simulink model "networkanalyzer"  (R2012b)
settings: Solver=ode3  SolverMode=SingleTasking  StartTime=0.0  StopTime=50000  RelTol=1e-3
libraries: xbsIndex_r4 x1097, casper_library_flow_control x33, casper_library_misc x21, xps_library x10
(part 5 of 8)

== system networkanalyzer/DFTMem2/MemRecord ==
  Start : Inport
  DataIn : Inport  Port=2
  WE : Inport  Port=3
  Constant6 : xbsIndex_r4/Constant  const=16383  gui_display_data_type=Fixed-point  arith_type=Unsigned  n_bits=14  bin_pt=0  preci_type=Single  exp_width=8  frac_width=24  explicit_period=off  period=1  equ=P=C  opselect=C  inp2=PCIN>>17  opr=+  inp1=P  carry=CIN  dbl_ovrd=off  block_type=constant
  Delay{,1..3} (4 alike) : xbsIndex_r4/Delay  rst=off  infoeditControl=Selection of Reset will increase slice count due to use of real FFs and instead of SRLs  en=off  latency=1  dbl_ovrd=off  reg_retiming=off  block_type=delay
  Gateway Out{1..6} (6 alike) : xbsIndex_r4/Gateway Out  inherit_from_input=off  hdl_port=off  timing_constraint=None  locs_specified=off  LOCs={}  UseAsDAC=off  DACChannel='1'  block_type=gatewayout
  Logical : xbsIndex_r4/Logical  logical_function=AND  inputs=2  en=off  latency=0  precision=Full  arith_type=Unsigned  n_bits=16  bin_pt=0  align_bp=on  dbl_ovrd=off  block_type=logical
  MCode : xbsIndex_r4/MCode  mfname=viewmemcontrol  explicit_period=on  period=1  inputsTable={'boundInpExpr'=>['start','endcnt','state'],'inputs'=>['start','endcnt','state']}  outputsTable={'outputs'=>['cnten','cntrst','nextstate'],'suppressOut'=>['off','off','off']}  dbl_ovrd=off  enable_stdout=on  enable_debug=off  suppress_output=on  defparams={'start',start,'endcnt',endcnt,'state',state}  hide_port_list={}  block_type=mcode
  Register : xbsIndex_r4/Register  init=0  rst=off  en=off  dbl_ovrd=off  block_type=register
  Relational : xbsIndex_r4/Relational  mode=a=b  en=off  latency=0  dbl_ovrd=off  block_type=relational
  Shared BRAM : Subsystem  Tag=xps:bram  AncestorBlock=xps_library/Shared BRAM  mask{arith_type=Unsigned, addr_width=14, data_width=32, reg_prim_output=off, reg_core_output=off, optimization=Minimum_Area, data_bin_pt=0, init_vals=[0:2^10-1], sample_rate=1}
      mask prompts: arith_type "Output Data Type"; addr_width "Address width"; data_width "Data Width"; reg_prim_output "Register Primitive Output"; reg_core_output "Register Core Output"; data_bin_pt "Data Binary Point"; init_vals "Initial values (simulation only)"; sample_rate "Sample rate"
      mask init:
      | shared_bram_mask;
      mask TypeOptions arith_type: Unsigned | Signed  (2's comp)
      mask TypeOptions data_width: 8 | 16 | 32 | 64 | 128
      mask TypeOptions optimization: Minimum_Area | Low_Power
  Terminator13 : Terminator
  memrecordscope : Scope  NumInputPorts=8
      settings: YMin=0~-5~-5~-5~-5~-5~-5~-5  YMax=300000~5~5~5~5~5~5~5  MaxDataPoints=10000
  spect_cnt : xbsIndex_r4/Counter  cnt_type=Free Running  cnt_to=Inf  operation=Up  start_count=0  cnt_by_val=1  arith_type=Unsigned  n_bits=14  bin_pt=0  load_pin=off  rst=on  en=on  explicit_period=on  period=1  dbl_ovrd=off  use_behavioral_HDL=off  implementation=Fabric  use_rpm=off  block_type=counter
  memDone : Outport
  wires:
  DataIn/1 -> Delay3/1
  Start/1 -> Gateway Out1/1, MCode/1
  spect_cnt/1 -> Relational/2, Gateway Out3/1, Delay1/1
  Delay/1 -> Terminator13/1
  Constant6/1 -> Relational/1
  MCode/2 -> spect_cnt/1
  Relational/1 -> Gateway Out6/1, memDone/1, MCode/2
  Register/1 -> MCode/3, Gateway Out2/1
  MCode/3 -> Register/1
  MCode/1 -> Logical/1
  Logical/1 -> Gateway Out4/1, Delay2/1, spect_cnt/2
  WE/1 -> Logical/2
  Gateway Out5/1 -> memrecordscope/1
  Gateway Out1/1 -> memrecordscope/2
  Gateway Out2/1 -> memrecordscope/3
  Gateway Out3/1 -> memrecordscope/4
  Gateway Out4/1 -> memrecordscope/5
  Gateway Out6/1 -> memrecordscope/6
  Delay1/1 -> Shared BRAM/1(addr)
  Delay3/1 -> Shared BRAM/2(data_in)
  Delay2/1 -> Shared BRAM/3(we)
  Shared BRAM/1(data_out) -> Gateway Out5/1, Delay/1

== system networkanalyzer/DFTMem3/MemRecord ==
  Start : Inport
  DataIn : Inport  Port=2
  WE : Inport  Port=3
  Constant6 : xbsIndex_r4/Constant  const=16383  gui_display_data_type=Fixed-point  arith_type=Unsigned  n_bits=14  bin_pt=0  preci_type=Single  exp_width=8  frac_width=24  explicit_period=off  period=1  equ=P=C  opselect=C  inp2=PCIN>>17  opr=+  inp1=P  carry=CIN  dbl_ovrd=off  block_type=constant
  Delay{,1..3} (4 alike) : xbsIndex_r4/Delay  rst=off  infoeditControl=Selection of Reset will increase slice count due to use of real FFs and instead of SRLs  en=off  latency=1  dbl_ovrd=off  reg_retiming=off  block_type=delay
  Gateway Out{1..6} (6 alike) : xbsIndex_r4/Gateway Out  inherit_from_input=off  hdl_port=off  timing_constraint=None  locs_specified=off  LOCs={}  UseAsDAC=off  DACChannel='1'  block_type=gatewayout
  Logical : xbsIndex_r4/Logical  logical_function=AND  inputs=2  en=off  latency=0  precision=Full  arith_type=Unsigned  n_bits=16  bin_pt=0  align_bp=on  dbl_ovrd=off  block_type=logical
  MCode : xbsIndex_r4/MCode  mfname=viewmemcontrol  explicit_period=on  period=1  inputsTable={'boundInpExpr'=>['start','endcnt','state'],'inputs'=>['start','endcnt','state']}  outputsTable={'outputs'=>['cnten','cntrst','nextstate'],'suppressOut'=>['off','off','off']}  dbl_ovrd=off  enable_stdout=on  enable_debug=off  suppress_output=on  defparams={'start',start,'endcnt',endcnt,'state',state}  hide_port_list={}  block_type=mcode
  Register : xbsIndex_r4/Register  init=0  rst=off  en=off  dbl_ovrd=off  block_type=register
  Relational : xbsIndex_r4/Relational  mode=a=b  en=off  latency=0  dbl_ovrd=off  block_type=relational
  Shared BRAM : Subsystem  Tag=xps:bram  AncestorBlock=xps_library/Shared BRAM  mask{arith_type=Unsigned, addr_width=14, data_width=32, reg_prim_output=off, reg_core_output=off, optimization=Minimum_Area, data_bin_pt=0, init_vals=[0:2^10-1], sample_rate=1}
      mask prompts: arith_type "Output Data Type"; addr_width "Address width"; data_width "Data Width"; reg_prim_output "Register Primitive Output"; reg_core_output "Register Core Output"; data_bin_pt "Data Binary Point"; init_vals "Initial values (simulation only)"; sample_rate "Sample rate"
      mask init:
      | shared_bram_mask;
      mask TypeOptions arith_type: Unsigned | Signed  (2's comp)
      mask TypeOptions data_width: 8 | 16 | 32 | 64 | 128
      mask TypeOptions optimization: Minimum_Area | Low_Power
  Terminator13 : Terminator
  memrecordscope : Scope  NumInputPorts=8
      settings: YMin=0~-5~-5~-5~-5~-5~-5~-5  YMax=300000~5~5~5~5~5~5~5  MaxDataPoints=10000
  spect_cnt : xbsIndex_r4/Counter  cnt_type=Free Running  cnt_to=Inf  operation=Up  start_count=0  cnt_by_val=1  arith_type=Unsigned  n_bits=14  bin_pt=0  load_pin=off  rst=on  en=on  explicit_period=on  period=1  dbl_ovrd=off  use_behavioral_HDL=off  implementation=Fabric  use_rpm=off  block_type=counter
  memDone : Outport
  wires:
  DataIn/1 -> Delay3/1
  Start/1 -> Gateway Out1/1, MCode/1
  spect_cnt/1 -> Relational/2, Gateway Out3/1, Delay1/1
  Delay/1 -> Terminator13/1
  Constant6/1 -> Relational/1
  MCode/2 -> spect_cnt/1
  Relational/1 -> Gateway Out6/1, memDone/1, MCode/2
  Register/1 -> MCode/3, Gateway Out2/1
  MCode/3 -> Register/1
  MCode/1 -> Logical/1
  Logical/1 -> Gateway Out4/1, Delay2/1, spect_cnt/2
  WE/1 -> Logical/2
  Gateway Out5/1 -> memrecordscope/1
  Gateway Out1/1 -> memrecordscope/2
  Gateway Out2/1 -> memrecordscope/3
  Gateway Out3/1 -> memrecordscope/4
  Gateway Out4/1 -> memrecordscope/5
  Gateway Out6/1 -> memrecordscope/6
  Delay1/1 -> Shared BRAM/1(addr)
  Delay3/1 -> Shared BRAM/2(data_in)
  Delay2/1 -> Shared BRAM/3(we)
  Shared BRAM/1(data_out) -> Gateway Out5/1, Delay/1

== system networkanalyzer/DFTMem4/MemRecord ==
  Start : Inport
  DataIn : Inport  Port=2
  WE : Inport  Port=3
  Constant6 : xbsIndex_r4/Constant  const=16383  gui_display_data_type=Fixed-point  arith_type=Unsigned  n_bits=14  bin_pt=0  preci_type=Single  exp_width=8  frac_width=24  explicit_period=off  period=1  equ=P=C  opselect=C  inp2=PCIN>>17  opr=+  inp1=P  carry=CIN  dbl_ovrd=off  block_type=constant
  Delay{,1..3} (4 alike) : xbsIndex_r4/Delay  rst=off  infoeditControl=Selection of Reset will increase slice count due to use of real FFs and instead of SRLs  en=off  latency=1  dbl_ovrd=off  reg_retiming=off  block_type=delay
  Gateway Out{1..6} (6 alike) : xbsIndex_r4/Gateway Out  inherit_from_input=off  hdl_port=off  timing_constraint=None  locs_specified=off  LOCs={}  UseAsDAC=off  DACChannel='1'  block_type=gatewayout
  Logical : xbsIndex_r4/Logical  logical_function=AND  inputs=2  en=off  latency=0  precision=Full  arith_type=Unsigned  n_bits=16  bin_pt=0  align_bp=on  dbl_ovrd=off  block_type=logical
  MCode : xbsIndex_r4/MCode  mfname=viewmemcontrol  explicit_period=on  period=1  inputsTable={'boundInpExpr'=>['start','endcnt','state'],'inputs'=>['start','endcnt','state']}  outputsTable={'outputs'=>['cnten','cntrst','nextstate'],'suppressOut'=>['off','off','off']}  dbl_ovrd=off  enable_stdout=on  enable_debug=off  suppress_output=on  defparams={'start',start,'endcnt',endcnt,'state',state}  hide_port_list={}  block_type=mcode
  Register : xbsIndex_r4/Register  init=0  rst=off  en=off  dbl_ovrd=off  block_type=register
  Relational : xbsIndex_r4/Relational  mode=a=b  en=off  latency=0  dbl_ovrd=off  block_type=relational
  Shared BRAM : Subsystem  Tag=xps:bram  AncestorBlock=xps_library/Shared BRAM  mask{arith_type=Unsigned, addr_width=14, data_width=32, reg_prim_output=off, reg_core_output=off, optimization=Minimum_Area, data_bin_pt=0, init_vals=[0:2^10-1], sample_rate=1}
      mask prompts: arith_type "Output Data Type"; addr_width "Address width"; data_width "Data Width"; reg_prim_output "Register Primitive Output"; reg_core_output "Register Core Output"; data_bin_pt "Data Binary Point"; init_vals "Initial values (simulation only)"; sample_rate "Sample rate"
      mask init:
      | shared_bram_mask;
      mask TypeOptions arith_type: Unsigned | Signed  (2's comp)
      mask TypeOptions data_width: 8 | 16 | 32 | 64 | 128
      mask TypeOptions optimization: Minimum_Area | Low_Power
  Terminator13 : Terminator
  memrecordscope : Scope  NumInputPorts=8
      settings: YMin=0~-5~-5~-5~-5~-5~-5~-5  YMax=300000~5~5~5~5~5~5~5  MaxDataPoints=10000
  spect_cnt : xbsIndex_r4/Counter  cnt_type=Free Running  cnt_to=Inf  operation=Up  start_count=0  cnt_by_val=1  arith_type=Unsigned  n_bits=14  bin_pt=0  load_pin=off  rst=on  en=on  explicit_period=on  period=1  dbl_ovrd=off  use_behavioral_HDL=off  implementation=Fabric  use_rpm=off  block_type=counter
  memDone : Outport
  wires:
  DataIn/1 -> Delay3/1
  Start/1 -> Gateway Out1/1, MCode/1
  spect_cnt/1 -> Relational/2, Gateway Out3/1, Delay1/1
  Delay/1 -> Terminator13/1
  Constant6/1 -> Relational/1
  MCode/2 -> spect_cnt/1
  Relational/1 -> Gateway Out6/1, memDone/1, MCode/2
  Register/1 -> MCode/3, Gateway Out2/1
  MCode/3 -> Register/1
  MCode/1 -> Logical/1
  Logical/1 -> Gateway Out4/1, Delay2/1, spect_cnt/2
  WE/1 -> Logical/2
  Gateway Out5/1 -> memrecordscope/1
  Gateway Out1/1 -> memrecordscope/2
  Gateway Out2/1 -> memrecordscope/3
  Gateway Out3/1 -> memrecordscope/4
  Gateway Out4/1 -> memrecordscope/5
  Gateway Out6/1 -> memrecordscope/6
  Delay1/1 -> Shared BRAM/1(addr)
  Delay3/1 -> Shared BRAM/2(data_in)
  Delay2/1 -> Shared BRAM/3(we)
  Shared BRAM/1(data_out) -> Gateway Out5/1, Delay/1

== system networkanalyzer/Stack4_/RegAddr ==
  Data : Inport
  Addr : Inport  Port=2
  WE : Inport  Port=3
  Constant : xbsIndex_r4/Constant  const=1  gui_display_data_type=Fixed-point  arith_type=Unsigned  n_bits=2  bin_pt=0  preci_type=Single  exp_width=8  frac_width=24  explicit_period=off  period=1  equ=P=C  opselect=C  inp2=PCIN>>17  opr=+  inp1=P  carry=CIN  dbl_ovrd=off  block_type=constant
  Logical1 : xbsIndex_r4/Logical  logical_function=AND  inputs=2  en=off  latency=0  precision=Full  arith_type=Unsigned  n_bits=16  bin_pt=0  align_bp=on  dbl_ovrd=off  block_type=logical
  Register : xbsIndex_r4/Register  init=0  rst=off  en=on  dbl_ovrd=off  block_type=register
  Relational : xbsIndex_r4/Relational  mode=a=b  en=off  latency=0  dbl_ovrd=off  block_type=relational
  DataOut : Outport
  wires:
  Logical1/1 -> Register/2
  Register/1 -> DataOut/1
  Data/1 -> Register/1
  WE/1 -> Logical1/2
  Relational/1 -> Logical1/1
  Constant/1 -> Relational/1
  Addr/1 -> Relational/2

== system networkanalyzer/Stack4_/RegAddr1 ==
  Data : Inport
  Addr : Inport  Port=2
  WE : Inport  Port=3
  Constant : xbsIndex_r4/Constant  const=2  gui_display_data_type=Fixed-point  arith_type=Unsigned  n_bits=2  bin_pt=0  preci_type=Single  exp_width=8  frac_width=24  explicit_period=off  period=1  equ=P=C  opselect=C  inp2=PCIN>>17  opr=+  inp1=P  carry=CIN  dbl_ovrd=off  block_type=constant
  Logical1 : xbsIndex_r4/Logical  logical_function=AND  inputs=2  en=off  latency=0  precision=Full  arith_type=Unsigned  n_bits=16  bin_pt=0  align_bp=on  dbl_ovrd=off  block_type=logical
  Register : xbsIndex_r4/Register  init=0  rst=off  en=on  dbl_ovrd=off  block_type=register
  Relational : xbsIndex_r4/Relational  mode=a=b  en=off  latency=0  dbl_ovrd=off  block_type=relational
  DataOut : Outport
  wires:
  Logical1/1 -> Register/2
  Register/1 -> DataOut/1
  Data/1 -> Register/1
  WE/1 -> Logical1/2
  Relational/1 -> Logical1/1
  Constant/1 -> Relational/1
  Addr/1 -> Relational/2

== system networkanalyzer/Stack4_/RegAddr2 ==
  Data : Inport
  Addr : Inport  Port=2
  WE : Inport  Port=3
  Constant : xbsIndex_r4/Constant  const=0  gui_display_data_type=Fixed-point  arith_type=Unsigned  n_bits=2  bin_pt=0  preci_type=Single  exp_width=8  frac_width=24  explicit_period=off  period=1  equ=P=C  opselect=C  inp2=PCIN>>17  opr=+  inp1=P  carry=CIN  dbl_ovrd=off  block_type=constant
  Logical1 : xbsIndex_r4/Logical  logical_function=AND  inputs=2  en=off  latency=0  precision=Full  arith_type=Unsigned  n_bits=16  bin_pt=0  align_bp=on  dbl_ovrd=off  block_type=logical
  Register : xbsIndex_r4/Register  init=0  rst=off  en=on  dbl_ovrd=off  block_type=register
  Relational : xbsIndex_r4/Relational  mode=a=b  en=off  latency=0  dbl_ovrd=off  block_type=relational
  DataOut : Outport
  wires:
  Logical1/1 -> Register/2
  Register/1 -> DataOut/1
  Data/1 -> Register/1
  WE/1 -> Logical1/2
  Relational/1 -> Logical1/1
  Constant/1 -> Relational/1
  Addr/1 -> Relational/2

== system networkanalyzer/Stack4_/RegAddr3 ==
  Data : Inport
  Addr : Inport  Port=2
  WE : Inport  Port=3
  Constant : xbsIndex_r4/Constant  const=3  gui_display_data_type=Fixed-point  arith_type=Unsigned  n_bits=2  bin_pt=0  preci_type=Single  exp_width=8  frac_width=24  explicit_period=off  period=1  equ=P=C  opselect=C  inp2=PCIN>>17  opr=+  inp1=P  carry=CIN  dbl_ovrd=off  block_type=constant
  Logical1 : xbsIndex_r4/Logical  logical_function=AND  inputs=2  en=off  latency=0  precision=Full  arith_type=Unsigned  n_bits=16  bin_pt=0  align_bp=on  dbl_ovrd=off  block_type=logical
  Register : xbsIndex_r4/Register  init=0  rst=off  en=on  dbl_ovrd=off  block_type=register
  Relational : xbsIndex_r4/Relational  mode=a=b  en=off  latency=0  dbl_ovrd=off  block_type=relational
  DataOut : Outport
  wires:
  Logical1/1 -> Register/2
  Register/1 -> DataOut/1
  Data/1 -> Register/1
  WE/1 -> Logical1/2
  Relational/1 -> Logical1/1
  Constant/1 -> Relational/1
  Addr/1 -> Relational/2

== system networkanalyzer/Stack4_/updownCnt ==
  Dec : Inport
  Inc : Inport  Port=2
  Rst : Inport  Port=3
  AddSub : xbsIndex_r4/AddSub  mode=Addition  use_carryin=off  use_carryout=off  en=off  latency=0  precision=User Defined  arith_type=Unsigned  n_bits=2  bin_pt=0  quantization=Truncate  overflow=Wrap  dbl_ovrd=off  use_behavioral_HDL=off  hw_selection=Fabric  pipelined=off  block_type=addsub
  AddSub1 : xbsIndex_r4/AddSub  mode=Subtraction  use_carryin=off  use_carryout=off  en=off  latency=0  precision=User Defined  arith_type=Unsigned  n_bits=2  bin_pt=0  quantization=Truncate  overflow=Wrap  dbl_ovrd=off  use_behavioral_HDL=off  hw_selection=Fabric  pipelined=off  block_type=addsub
  Constant1 : xbsIndex_r4/Constant  const=1  gui_display_data_type=Fixed-point  arith_type=Unsigned  n_bits=2  bin_pt=0  preci_type=Single  exp_width=8  frac_width=24  explicit_period=off  period=1  equ=P=C  opselect=C  inp2=PCIN>>17  opr=+  inp1=P  carry=CIN  dbl_ovrd=off  block_type=constant
  Gateway Out{1..5,7} (6 alike) : xbsIndex_r4/Gateway Out  inherit_from_input=off  hdl_port=off  timing_constraint=None  locs_specified=off  LOCs={}  UseAsDAC=off  DACChannel='1'  block_type=gatewayout
  Logical : xbsIndex_r4/Logical  logical_function=OR  inputs=2  en=off  latency=0  precision=Full  arith_type=Unsigned  n_bits=16  bin_pt=0  align_bp=on  dbl_ovrd=off  block_type=logical
  Mux : xbsIndex_r4/Mux  inputs=2  en=off  latency=0  precision=User Defined  arith_type=Unsigned  n_bits=2  bin_pt=0  quantization=Truncate  overflow=Wrap  dbl_ovrd=off  block_type=mux
  Register1 : xbsIndex_r4/Register  init=0  rst=on  en=on  dbl_ovrd=off  block_type=register
  Scope1 : Scope  NumInputPorts=8
      settings: YMin=0~-5~-5~-5~-5~-5~-5~-5  YMax=300000~5~5~5~5~5~5~5  SaveName=ScopeData13  MaxDataPoints=10000
  Out : Outport
  wires:
  Register1/1 -> AddSub/2, AddSub1/1, Gateway Out2/1, Out/1
  Rst/1 -> Register1/2
  Mux/1 -> Register1/1, Gateway Out3/1
  Constant1/1 -> AddSub1/2, AddSub/1
  AddSub/1 -> Mux/2, Gateway Out4/1
  AddSub1/1 -> Mux/3, Gateway Out5/1
  Dec/1 -> Gateway Out1/1, Logical/2, Mux/1
  Logical/1 -> Register1/3
  Inc/1 -> Gateway Out7/1, Logical/1
  Gateway Out7/1 -> Scope1/1
  Gateway Out1/1 -> Scope1/2
  Gateway Out2/1 -> Scope1/3
  Gateway Out3/1 -> Scope1/4
  Gateway Out4/1 -> Scope1/5
  Gateway Out5/1 -> Scope1/6

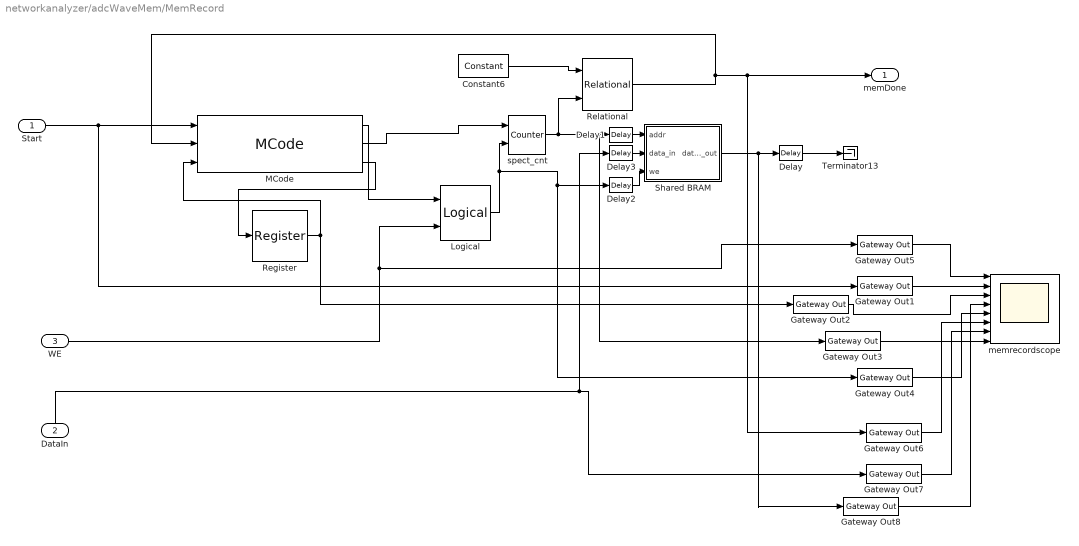
== system networkanalyzer/adcWaveMem/MemRecord ==
  Start : Inport
  DataIn : Inport  Port=2
  WE : Inport  Port=3
  Constant6 : xbsIndex_r4/Constant  const=4095  gui_display_data_type=Fixed-point  arith_type=Unsigned  n_bits=12  bin_pt=0  preci_type=Single  exp_width=8  frac_width=24  explicit_period=off  period=1  equ=P=C  opselect=C  inp2=PCIN>>17  opr=+  inp1=P  carry=CIN  dbl_ovrd=off  block_type=constant
  Delay{,1..3} (4 alike) : xbsIndex_r4/Delay  rst=off  infoeditControl=Selection of Reset will increase slice count due to use of real FFs and instead of SRLs  en=off  latency=1  dbl_ovrd=off  reg_retiming=off  block_type=delay
  Gateway Out{1..8} (8 alike) : xbsIndex_r4/Gateway Out  inherit_from_input=off  hdl_port=off  timing_constraint=None  locs_specified=off  LOCs={}  UseAsDAC=off  DACChannel='1'  block_type=gatewayout
  Logical : xbsIndex_r4/Logical  logical_function=AND  inputs=2  en=off  latency=0  precision=Full  arith_type=Unsigned  n_bits=16  bin_pt=0  align_bp=on  dbl_ovrd=off  block_type=logical
  MCode : xbsIndex_r4/MCode  mfname=viewmemcontrol  explicit_period=on  period=1  inputsTable={'boundInpExpr'=>['start','endcnt','state'],'inputs'=>['start','endcnt','state']}  outputsTable={'outputs'=>['cnten','cntrst','nextstate'],'suppressOut'=>['off','off','off']}  dbl_ovrd=off  enable_stdout=on  enable_debug=off  suppress_output=on  defparams={'start',start,'endcnt',endcnt,'state',state}  hide_port_list={}  block_type=mcode
  Register : xbsIndex_r4/Register  init=0  rst=off  en=off  dbl_ovrd=off  block_type=register
  Relational : xbsIndex_r4/Relational  mode=a=b  en=off  latency=0  dbl_ovrd=off  block_type=relational
  Shared BRAM : Subsystem  Tag=xps:bram  AncestorBlock=xps_library/Shared BRAM  mask{arith_type=Unsigned, addr_width=12, data_width=32, reg_prim_output=off, reg_core_output=off, optimization=Minimum_Area, data_bin_pt=0, init_vals=[0:2^10-1], sample_rate=1}
      mask prompts: arith_type "Output Data Type"; addr_width "Address width"; data_width "Data Width"; reg_prim_output "Register Primitive Output"; reg_core_output "Register Core Output"; data_bin_pt "Data Binary Point"; init_vals "Initial values (simulation only)"; sample_rate "Sample rate"
      mask init:
      | shared_bram_mask;
      mask TypeOptions arith_type: Unsigned | Signed  (2's comp)
      mask TypeOptions data_width: 8 | 16 | 32 | 64 | 128
      mask TypeOptions optimization: Minimum_Area | Low_Power
  Terminator13 : Terminator
  memrecordscope : Scope  NumInputPorts=8
      settings: YMin=0~-5~-5~-5~-5~-5~-5~-5  YMax=300000~5~5~5~5~5~5~5  MaxDataPoints=10000
  spect_cnt : xbsIndex_r4/Counter  cnt_type=Free Running  cnt_to=Inf  operation=Up  start_count=0  cnt_by_val=1  arith_type=Unsigned  n_bits=12  bin_pt=0  load_pin=off  rst=on  en=on  explicit_period=on  period=1  dbl_ovrd=off  use_behavioral_HDL=off  implementation=Fabric  use_rpm=off  block_type=counter
  memDone : Outport
  wires:
  DataIn/1 -> Gateway Out7/1, Delay3/1
  Start/1 -> Gateway Out1/1, MCode/1
  spect_cnt/1 -> Relational/2, Gateway Out3/1, Delay1/1
  Delay/1 -> Terminator13/1
  Constant6/1 -> Relational/1
  MCode/2 -> spect_cnt/1
  Relational/1 -> Gateway Out6/1, memDone/1, MCode/2
  Register/1 -> MCode/3, Gateway Out2/1
  MCode/3 -> Register/1
  MCode/1 -> Logical/1
  Logical/1 -> Gateway Out4/1, Delay2/1, spect_cnt/2
  WE/1 -> Gateway Out5/1, Logical/2
  Gateway Out5/1 -> memrecordscope/1
  Gateway Out1/1 -> memrecordscope/2
  Gateway Out2/1 -> memrecordscope/3
  Gateway Out3/1 -> memrecordscope/4
  Gateway Out4/1 -> memrecordscope/5
  Gateway Out6/1 -> memrecordscope/6
  Delay1/1 -> Shared BRAM/1(addr)
  Delay3/1 -> Shared BRAM/2(data_in)
  Delay2/1 -> Shared BRAM/3(we)
  Shared BRAM/1(data_out) -> Gateway Out8/1, Delay/1
  Gateway Out7/1 -> memrecordscope/7
  Gateway Out8/1 -> memrecordscope/8

== system networkanalyzer/adcWaveMem1/MemRecord ==
  Start : Inport
  DataIn : Inport  Port=2
  WE : Inport  Port=3
  Constant6 : xbsIndex_r4/Constant  const=4095  gui_display_data_type=Fixed-point  arith_type=Unsigned  n_bits=12  bin_pt=0  preci_type=Single  exp_width=8  frac_width=24  explicit_period=off  period=1  equ=P=C  opselect=C  inp2=PCIN>>17  opr=+  inp1=P  carry=CIN  dbl_ovrd=off  block_type=constant
  Delay{,1..3} (4 alike) : xbsIndex_r4/Delay  rst=off  infoeditControl=Selection of Reset will increase slice count due to use of real FFs and instead of SRLs  en=off  latency=1  dbl_ovrd=off  reg_retiming=off  block_type=delay
  Gateway Out{1..8} (8 alike) : xbsIndex_r4/Gateway Out  inherit_from_input=off  hdl_port=off  timing_constraint=None  locs_specified=off  LOCs={}  UseAsDAC=off  DACChannel='1'  block_type=gatewayout
  Logical : xbsIndex_r4/Logical  logical_function=AND  inputs=2  en=off  latency=0  precision=Full  arith_type=Unsigned  n_bits=16  bin_pt=0  align_bp=on  dbl_ovrd=off  block_type=logical
  MCode : xbsIndex_r4/MCode  mfname=viewmemcontrol  explicit_period=on  period=1  inputsTable={'boundInpExpr'=>['start','endcnt','state'],'inputs'=>['start','endcnt','state']}  outputsTable={'outputs'=>['cnten','cntrst','nextstate'],'suppressOut'=>['off','off','off']}  dbl_ovrd=off  enable_stdout=on  enable_debug=off  suppress_output=on  defparams={'start',start,'endcnt',endcnt,'state',state}  hide_port_list={}  block_type=mcode
  Register : xbsIndex_r4/Register  init=0  rst=off  en=off  dbl_ovrd=off  block_type=register
  Relational : xbsIndex_r4/Relational  mode=a=b  en=off  latency=0  dbl_ovrd=off  block_type=relational
  Shared BRAM : Subsystem  Tag=xps:bram  AncestorBlock=xps_library/Shared BRAM  mask{arith_type=Unsigned, addr_width=12, data_width=32, reg_prim_output=off, reg_core_output=off, optimization=Minimum_Area, data_bin_pt=0, init_vals=[0:2^10-1], sample_rate=1}
      mask prompts: arith_type "Output Data Type"; addr_width "Address width"; data_width "Data Width"; reg_prim_output "Register Primitive Output"; reg_core_output "Register Core Output"; data_bin_pt "Data Binary Point"; init_vals "Initial values (simulation only)"; sample_rate "Sample rate"
      mask init:
      | shared_bram_mask;
      mask TypeOptions arith_type: Unsigned | Signed  (2's comp)
      mask TypeOptions data_width: 8 | 16 | 32 | 64 | 128
      mask TypeOptions optimization: Minimum_Area | Low_Power
  Terminator13 : Terminator
  memrecordscope : Scope  NumInputPorts=8
      settings: YMin=0~-5~-5~-5~-5~-5~-5~-5  YMax=300000~5~5~5~5~5~5~5  MaxDataPoints=10000
  spect_cnt : xbsIndex_r4/Counter  cnt_type=Free Running  cnt_to=Inf  operation=Up  start_count=0  cnt_by_val=1  arith_type=Unsigned  n_bits=12  bin_pt=0  load_pin=off  rst=on  en=on  explicit_period=on  period=1  dbl_ovrd=off  use_behavioral_HDL=off  implementation=Fabric  use_rpm=off  block_type=counter
  memDone : Outport
  wires:
  DataIn/1 -> Gateway Out7/1, Delay3/1
  Start/1 -> Gateway Out1/1, MCode/1
  spect_cnt/1 -> Relational/2, Gateway Out3/1, Delay1/1
  Delay/1 -> Terminator13/1
  Constant6/1 -> Relational/1
  MCode/2 -> spect_cnt/1
  Relational/1 -> Gateway Out6/1, memDone/1, MCode/2
  Register/1 -> MCode/3, Gateway Out2/1
  MCode/3 -> Register/1
  MCode/1 -> Logical/1
  Logical/1 -> Gateway Out4/1, Delay2/1, spect_cnt/2
  WE/1 -> Gateway Out5/1, Logical/2
  Gateway Out5/1 -> memrecordscope/1
  Gateway Out1/1 -> memrecordscope/2
  Gateway Out2/1 -> memrecordscope/3
  Gateway Out3/1 -> memrecordscope/4
  Gateway Out4/1 -> memrecordscope/5
  Gateway Out6/1 -> memrecordscope/6
  Delay1/1 -> Shared BRAM/1(addr)
  Delay3/1 -> Shared BRAM/2(data_in)
  Delay2/1 -> Shared BRAM/3(we)
  Shared BRAM/1(data_out) -> Gateway Out8/1, Delay/1
  Gateway Out7/1 -> memrecordscope/7
  Gateway Out8/1 -> memrecordscope/8

== system networkanalyzer/adcWaveMem2/MemRecord ==
  Start : Inport
  DataIn : Inport  Port=2
  WE : Inport  Port=3
  Constant6 : xbsIndex_r4/Constant  const=4095  gui_display_data_type=Fixed-point  arith_type=Unsigned  n_bits=12  bin_pt=0  preci_type=Single  exp_width=8  frac_width=24  explicit_period=off  period=1  equ=P=C  opselect=C  inp2=PCIN>>17  opr=+  inp1=P  carry=CIN  dbl_ovrd=off  block_type=constant
  Delay{,1..3} (4 alike) : xbsIndex_r4/Delay  rst=off  infoeditControl=Selection of Reset will increase slice count due to use of real FFs and instead of SRLs  en=off  latency=1  dbl_ovrd=off  reg_retiming=off  block_type=delay
  Gateway Out{1..8} (8 alike) : xbsIndex_r4/Gateway Out  inherit_from_input=off  hdl_port=off  timing_constraint=None  locs_specified=off  LOCs={}  UseAsDAC=off  DACChannel='1'  block_type=gatewayout
  Logical : xbsIndex_r4/Logical  logical_function=AND  inputs=2  en=off  latency=0  precision=Full  arith_type=Unsigned  n_bits=16  bin_pt=0  align_bp=on  dbl_ovrd=off  block_type=logical
  MCode : xbsIndex_r4/MCode  mfname=viewmemcontrol  explicit_period=on  period=1  inputsTable={'boundInpExpr'=>['start','endcnt','state'],'inputs'=>['start','endcnt','state']}  outputsTable={'outputs'=>['cnten','cntrst','nextstate'],'suppressOut'=>['off','off','off']}  dbl_ovrd=off  enable_stdout=on  enable_debug=off  suppress_output=on  defparams={'start',start,'endcnt',endcnt,'state',state}  hide_port_list={}  block_type=mcode
  Register : xbsIndex_r4/Register  init=0  rst=off  en=off  dbl_ovrd=off  block_type=register
  Relational : xbsIndex_r4/Relational  mode=a=b  en=off  latency=0  dbl_ovrd=off  block_type=relational
  Shared BRAM : Subsystem  Tag=xps:bram  AncestorBlock=xps_library/Shared BRAM  mask{arith_type=Unsigned, addr_width=12, data_width=32, reg_prim_output=off, reg_core_output=off, optimization=Minimum_Area, data_bin_pt=0, init_vals=[0:2^10-1], sample_rate=1}
      mask prompts: arith_type "Output Data Type"; addr_width "Address width"; data_width "Data Width"; reg_prim_output "Register Primitive Output"; reg_core_output "Register Core Output"; data_bin_pt "Data Binary Point"; init_vals "Initial values (simulation only)"; sample_rate "Sample rate"
      mask init:
      | shared_bram_mask;
      mask TypeOptions arith_type: Unsigned | Signed  (2's comp)
      mask TypeOptions data_width: 8 | 16 | 32 | 64 | 128
      mask TypeOptions optimization: Minimum_Area | Low_Power
  Terminator13 : Terminator
  memrecordscope : Scope  NumInputPorts=8
      settings: YMin=0~-5~-5~-5~-5~-5~-5~-5  YMax=300000~5~5~5~5~5~5~5  MaxDataPoints=10000
  spect_cnt : xbsIndex_r4/Counter  cnt_type=Free Running  cnt_to=Inf  operation=Up  start_count=0  cnt_by_val=1  arith_type=Unsigned  n_bits=12  bin_pt=0  load_pin=off  rst=on  en=on  explicit_period=on  period=1  dbl_ovrd=off  use_behavioral_HDL=off  implementation=Fabric  use_rpm=off  block_type=counter
  memDone : Outport
  wires:
  DataIn/1 -> Gateway Out7/1, Delay3/1
  Start/1 -> Gateway Out1/1, MCode/1
  spect_cnt/1 -> Relational/2, Gateway Out3/1, Delay1/1
  Delay/1 -> Terminator13/1
  Constant6/1 -> Relational/1
  MCode/2 -> spect_cnt/1
  Relational/1 -> Gateway Out6/1, memDone/1, MCode/2
  Register/1 -> MCode/3, Gateway Out2/1
  MCode/3 -> Register/1
  MCode/1 -> Logical/1
  Logical/1 -> Gateway Out4/1, Delay2/1, spect_cnt/2
  WE/1 -> Gateway Out5/1, Logical/2
  Gateway Out5/1 -> memrecordscope/1
  Gateway Out1/1 -> memrecordscope/2
  Gateway Out2/1 -> memrecordscope/3
  Gateway Out3/1 -> memrecordscope/4
  Gateway Out4/1 -> memrecordscope/5
  Gateway Out6/1 -> memrecordscope/6
  Delay1/1 -> Shared BRAM/1(addr)
  Delay3/1 -> Shared BRAM/2(data_in)
  Delay2/1 -> Shared BRAM/3(we)
  Shared BRAM/1(data_out) -> Gateway Out8/1, Delay/1
  Gateway Out7/1 -> memrecordscope/7
  Gateway Out8/1 -> memrecordscope/8

== system networkanalyzer/adcWaveMem3/MemRecord ==
  Start : Inport
  DataIn : Inport  Port=2
  WE : Inport  Port=3
  Constant6 : xbsIndex_r4/Constant  const=4095  gui_display_data_type=Fixed-point  arith_type=Unsigned  n_bits=12  bin_pt=0  preci_type=Single  exp_width=8  frac_width=24  explicit_period=off  period=1  equ=P=C  opselect=C  inp2=PCIN>>17  opr=+  inp1=P  carry=CIN  dbl_ovrd=off  block_type=constant
  Delay{,1..3} (4 alike) : xbsIndex_r4/Delay  rst=off  infoeditControl=Selection of Reset will increase slice count due to use of real FFs and instead of SRLs  en=off  latency=1  dbl_ovrd=off  reg_retiming=off  block_type=delay
  Gateway Out{1..8} (8 alike) : xbsIndex_r4/Gateway Out  inherit_from_input=off  hdl_port=off  timing_constraint=None  locs_specified=off  LOCs={}  UseAsDAC=off  DACChannel='1'  block_type=gatewayout
  Logical : xbsIndex_r4/Logical  logical_function=AND  inputs=2  en=off  latency=0  precision=Full  arith_type=Unsigned  n_bits=16  bin_pt=0  align_bp=on  dbl_ovrd=off  block_type=logical
  MCode : xbsIndex_r4/MCode  mfname=viewmemcontrol  explicit_period=on  period=1  inputsTable={'boundInpExpr'=>['start','endcnt','state'],'inputs'=>['start','endcnt','state']}  outputsTable={'outputs'=>['cnten','cntrst','nextstate'],'suppressOut'=>['off','off','off']}  dbl_ovrd=off  enable_stdout=on  enable_debug=off  suppress_output=on  defparams={'start',start,'endcnt',endcnt,'state',state}  hide_port_list={}  block_type=mcode
  Register : xbsIndex_r4/Register  init=0  rst=off  en=off  dbl_ovrd=off  block_type=register
  Relational : xbsIndex_r4/Relational  mode=a=b  en=off  latency=0  dbl_ovrd=off  block_type=relational
  Shared BRAM : Subsystem  Tag=xps:bram  AncestorBlock=xps_library/Shared BRAM  mask{arith_type=Unsigned, addr_width=12, data_width=32, reg_prim_output=off, reg_core_output=off, optimization=Minimum_Area, data_bin_pt=0, init_vals=[0:2^10-1], sample_rate=1}
      mask prompts: arith_type "Output Data Type"; addr_width "Address width"; data_width "Data Width"; reg_prim_output "Register Primitive Output"; reg_core_output "Register Core Output"; data_bin_pt "Data Binary Point"; init_vals "Initial values (simulation only)"; sample_rate "Sample rate"
      mask init:
      | shared_bram_mask;
      mask TypeOptions arith_type: Unsigned | Signed  (2's comp)
      mask TypeOptions data_width: 8 | 16 | 32 | 64 | 128
      mask TypeOptions optimization: Minimum_Area | Low_Power
  Terminator13 : Terminator
  memrecordscope : Scope  NumInputPorts=8
      settings: YMin=0~-5~-5~-5~-5~-5~-5~-5  YMax=300000~5~5~5~5~5~5~5  MaxDataPoints=10000
  spect_cnt : xbsIndex_r4/Counter  cnt_type=Free Running  cnt_to=Inf  operation=Up  start_count=0  cnt_by_val=1  arith_type=Unsigned  n_bits=12  bin_pt=0  load_pin=off  rst=on  en=on  explicit_period=on  period=1  dbl_ovrd=off  use_behavioral_HDL=off  implementation=Fabric  use_rpm=off  block_type=counter
  memDone : Outport
  wires:
  DataIn/1 -> Gateway Out7/1, Delay3/1
  Start/1 -> Gateway Out1/1, MCode/1
  spect_cnt/1 -> Relational/2, Gateway Out3/1, Delay1/1
  Delay/1 -> Terminator13/1
  Constant6/1 -> Relational/1
  MCode/2 -> spect_cnt/1
  Relational/1 -> Gateway Out6/1, memDone/1, MCode/2
  Register/1 -> MCode/3, Gateway Out2/1
  MCode/3 -> Register/1
  MCode/1 -> Logical/1
  Logical/1 -> Gateway Out4/1, Delay2/1, spect_cnt/2
  WE/1 -> Gateway Out5/1, Logical/2
  Gateway Out5/1 -> memrecordscope/1
  Gateway Out1/1 -> memrecordscope/2
  Gateway Out2/1 -> memrecordscope/3
  Gateway Out3/1 -> memrecordscope/4
  Gateway Out4/1 -> memrecordscope/5
  Gateway Out6/1 -> memrecordscope/6
  Delay1/1 -> Shared BRAM/1(addr)
  Delay3/1 -> Shared BRAM/2(data_in)
  Delay2/1 -> Shared BRAM/3(we)
  Shared BRAM/1(data_out) -> Gateway Out8/1, Delay/1
  Gateway Out7/1 -> memrecordscope/7
  Gateway Out8/1 -> memrecordscope/8

== system networkanalyzer/DFTMem1/MemRecord/Shared BRAM ==
  addr : Inport
  data_in : Inport  Port=2
  we : Inport  Port=3
  calc_add : Subsystem  mask{data_width=32, addr_width=14, sample_rate=sample_rate}
      mask prompts: data_width "data width"; addr_width "address width"; sample_rate "sample rate"
  convert_addr : xbsIndex_r4/Convert  gui_display_data_type=Fixed-point  arith_type=Unsigned  n_bits=addr_width  bin_pt=0  float_type=Single  exp_bits=8  fraction_bits=24  quantization=Truncate  overflow=Wrap  en=off  latency=0  dbl_ovrd=off  pipeline=off  block_type=convert
      settings: xl_area=[0, 0, 0, 0, 0, 0, 0]
  convert_din1 : xbsIndex_r4/Convert  gui_display_data_type=Fixed-point  arith_type=Unsigned  n_bits=32  bin_pt=0  float_type=Single  exp_bits=8  fraction_bits=24  quantization=Truncate  overflow=Wrap  en=off  latency=0  dbl_ovrd=off  pipeline=off  block_type=convert
      settings: xl_area=[0, 0, 0, 0, 0, 0, 0]
  convert_we : xbsIndex_r4/Convert  gui_display_data_type=Fixed-point  arith_type=Unsigned  n_bits=1  bin_pt=0  float_type=Single  exp_bits=8  fraction_bits=24  quantization=Truncate  overflow=Wrap  en=off  latency=0  dbl_ovrd=off  pipeline=off  block_type=convert
      settings: xl_area=[0, 0, 0, 0, 0, 0, 0]
  mem : Subsystem
  munge_in : Subsystem  AncestorBlock=casper_library_flow_control/munge  mask(munge){divisions=1, div_size=32, order=[0], arith_type_out=Unsigned, bin_pt_out=0}
      mask prompts: divisions "Number of divisions"; div_size "Division size (bits)"; order "Division packing order"; arith_type_out "Output arithmetic type"; bin_pt_out "Output binary point"
      mask help: Splits an input bus into the specified number of divisions and then recombines them in the order specified (most significant division = 0,least = number divisions-1)
      mask init:
      | munge_init(gcb, ...
      |     'divisions', divisions, ...
      |     'div_size', div_size, ...
      |     'order', order, ...
      |     'arith_type_out', arith_type_out, ...
      |     'bin_pt_out', bin_pt_out);
      settings: AttributesFormatString=|
      | split:32
      | join:0
      | Unsigned [32,0]
      mask TypeOptions arith_type_out: Unsigned | Signed  (2's comp) | Floating-point
  munge_out : Subsystem  AncestorBlock=casper_library_flow_control/munge  mask(munge){divisions=1, div_size=32, order=[0], arith_type_out=Unsigned, bin_pt_out=0}
      mask prompts: divisions "Number of divisions"; div_size "Division size (bits)"; order "Division packing order"; arith_type_out "Output arithmetic type"; bin_pt_out "Output binary point"
      mask help: Splits an input bus into the specified number of divisions and then recombines them in the order specified (most significant division = 0,least = number divisions-1)
      mask init:
      | munge_init(gcb, ...
      |     'divisions', divisions, ...
      |     'div_size', div_size, ...
      |     'order', order, ...
      |     'arith_type_out', arith_type_out, ...
      |     'bin_pt_out', bin_pt_out);
      settings: AttributesFormatString=|
      | split:32
      | join:0
      | Unsigned [32,0]
      mask TypeOptions arith_type_out: Unsigned | Signed  (2's comp) | Floating-point
  networkanalyzer_DFTMem1_MemRecord_Shared_BRAM_addr : xbsIndex_r4/Gateway Out  inherit_from_input=off  hdl_port=on  timing_constraint=None  locs_specified=off  LOCs={'A5','B9','A9','C1','A3','G6','E9','A6','A7','A8','B8','B1','B3','D9','B5','B4','B6','C2'}  UseAsDAC=off  DACChannel='1'  block_type=gatewayout
      settings: infoedit="Gateway out block.  Converts Xilinx fixed point inputs into ouputs of type Simulink integer, double, or fixed point.<P><P>Hardware notes:  In hardware these blocks become top level output ports or are discarded, depending on how they are configured."  xl_area=[0, 0, 0, 0, 0, 0, 0]  sginterface={'Nallatech'=>{'xdspkit'=>{'non_memory_mapped_port'=>'uprev_Shared_BRAM_addr'}},'Xilinx'=>{'jtaghwcosim'=>{'non_memory_mapped_port'=>'uprev_Shared_BRAM_addr'},'xdspkit'=>{'non_memory_mapped_port'=>'uprev_Shared_BRAM_addr'}}}
  networkanalyzer_DFTMem1_MemRecord_Shared_BRAM_data_in : xbsIndex_r4/Gateway Out  inherit_from_input=off  hdl_port=on  timing_constraint=None  locs_specified=off  LOCs={'B21','B22','A22','B23','B19','C19','A20','A21','A23','B24','A24','A25','E18','D18','C18','B18'}  UseAsDAC=off  DACChannel='1'  block_type=gatewayout
      settings: infoedit="Gateway out block.  Converts Xilinx fixed point inputs into ouputs of type Simulink integer, double, or fixed point.<P><P>Hardware notes:  In hardware these blocks become top level output ports or are discarded, depending on how they are configured."  xl_area=[0, 0, 0, 0, 0, 0, 0]  sginterface={'Nallatech'=>{'xdspkit'=>{'non_memory_mapped_port'=>'uprev_Shared_BRAM_data_in'}},'Xilinx'=>{'jtaghwcosim'=>{'non_memory_mapped_port'=>'uprev_Shared_BRAM_data_in'},'xdspkit'=>{'non_memory_mapped_port'=>'uprev_Shared_BRAM_data_in'}}}
  networkanalyzer_DFTMem1_MemRecord_Shared_BRAM_data_out : xbsIndex_r4/Gateway In  gui_display_data_type=Fixed-point  arith_type=Unsigned  n_bits=32  bin_pt=0  preci_type=Single  exp_width=8  frac_width=24  quantization=Truncate  overflow=Wrap  period=sample_rate  dbl_ovrd=off  timing_constraint=None  locs_specified=off  LOCs={}  UseAsADC=off  ADCChannel='1'  inherit_from_input=off  hdl_port=on  block_type=gatewayin
      settings: xl_area=[0, 0, 0, 0, 0, 0, 0]
  networkanalyzer_DFTMem1_MemRecord_Shared_BRAM_we : xbsIndex_r4/Gateway Out  inherit_from_input=off  hdl_port=on  timing_constraint=None  locs_specified=off  LOCs={'A14'}  UseAsDAC=off  DACChannel='1'  block_type=gatewayout
      settings: infoedit="Gateway out block.  Converts Xilinx fixed point inputs into ouputs of type Simulink integer, double, or fixed point.<P><P>Hardware notes:  In hardware these blocks become top level output ports or are discarded, depending on how they are configured."  xl_area=[0, 0, 0, 0, 0, 0, 0]
  data_out : Outport
  wires:
  convert_addr/1 -> networkanalyzer_DFTMem1_MemRecord_Shared_BRAM_addr/1
  convert_din1/1 -> networkanalyzer_DFTMem1_MemRecord_Shared_BRAM_data_in/1
  data_in/1 -> munge_in/1(din)
  calc_add/1(out) -> convert_addr/1
  networkanalyzer_DFTMem1_MemRecord_Shared_BRAM_we/1 -> mem/3(In3)
  networkanalyzer_DFTMem1_MemRecord_Shared_BRAM_data_in/1 -> mem/2(In2)
  networkanalyzer_DFTMem1_MemRecord_Shared_BRAM_addr/1 -> mem/1(In1)
  convert_we/1 -> networkanalyzer_DFTMem1_MemRecord_Shared_BRAM_we/1
  networkanalyzer_DFTMem1_MemRecord_Shared_BRAM_data_out/1 -> munge_out/1(din)
  mem/1(Out1) -> networkanalyzer_DFTMem1_MemRecord_Shared_BRAM_data_out/1
  addr/1 -> calc_add/1(in)
  we/1 -> convert_we/1
  munge_out/1(dout) -> data_out/1
  munge_in/1(dout) -> convert_din1/1

== system networkanalyzer/DFTMem2/MemRecord/Shared BRAM ==
  addr : Inport
  data_in : Inport  Port=2
  we : Inport  Port=3
  calc_add : Subsystem  mask{data_width=32, addr_width=14, sample_rate=sample_rate}
      mask prompts: data_width "data width"; addr_width "address width"; sample_rate "sample rate"
  convert_addr : xbsIndex_r4/Convert  gui_display_data_type=Fixed-point  arith_type=Unsigned  n_bits=addr_width  bin_pt=0  float_type=Single  exp_bits=8  fraction_bits=24  quantization=Truncate  overflow=Wrap  en=off  latency=0  dbl_ovrd=off  pipeline=off  block_type=convert
      settings: xl_area=[0, 0, 0, 0, 0, 0, 0]
  convert_din1 : xbsIndex_r4/Convert  gui_display_data_type=Fixed-point  arith_type=Unsigned  n_bits=32  bin_pt=0  float_type=Single  exp_bits=8  fraction_bits=24  quantization=Truncate  overflow=Wrap  en=off  latency=0  dbl_ovrd=off  pipeline=off  block_type=convert
      settings: xl_area=[0, 0, 0, 0, 0, 0, 0]
  convert_we : xbsIndex_r4/Convert  gui_display_data_type=Fixed-point  arith_type=Unsigned  n_bits=1  bin_pt=0  float_type=Single  exp_bits=8  fraction_bits=24  quantization=Truncate  overflow=Wrap  en=off  latency=0  dbl_ovrd=off  pipeline=off  block_type=convert
      settings: xl_area=[0, 0, 0, 0, 0, 0, 0]
  mem : Subsystem
  munge_in : Subsystem  AncestorBlock=casper_library_flow_control/munge  mask(munge){divisions=1, div_size=32, order=[0], arith_type_out=Unsigned, bin_pt_out=0}
      mask prompts: divisions "Number of divisions"; div_size "Division size (bits)"; order "Division packing order"; arith_type_out "Output arithmetic type"; bin_pt_out "Output binary point"
      mask help: Splits an input bus into the specified number of divisions and then recombines them in the order specified (most significant division = 0,least = number divisions-1)
      mask init:
      | munge_init(gcb, ...
      |     'divisions', divisions, ...
      |     'div_size', div_size, ...
      |     'order', order, ...
      |     'arith_type_out', arith_type_out, ...
      |     'bin_pt_out', bin_pt_out);
      settings: AttributesFormatString=|
      | split:32
      | join:0
      | Unsigned [32,0]
      mask TypeOptions arith_type_out: Unsigned | Signed  (2's comp) | Floating-point
  munge_out : Subsystem  AncestorBlock=casper_library_flow_control/munge  mask(munge){divisions=1, div_size=32, order=[0], arith_type_out=Unsigned, bin_pt_out=0}
      mask prompts: divisions "Number of divisions"; div_size "Division size (bits)"; order "Division packing order"; arith_type_out "Output arithmetic type"; bin_pt_out "Output binary point"
      mask help: Splits an input bus into the specified number of divisions and then recombines them in the order specified (most significant division = 0,least = number divisions-1)
      mask init:
      | munge_init(gcb, ...
      |     'divisions', divisions, ...
      |     'div_size', div_size, ...
      |     'order', order, ...
      |     'arith_type_out', arith_type_out, ...
      |     'bin_pt_out', bin_pt_out);
      settings: AttributesFormatString=|
      | split:32
      | join:0
      | Unsigned [32,0]
      mask TypeOptions arith_type_out: Unsigned | Signed  (2's comp) | Floating-point
  networkanalyzer_DFTMem2_MemRecord_Shared_BRAM_addr : xbsIndex_r4/Gateway Out  inherit_from_input=off  hdl_port=on  timing_constraint=None  locs_specified=off  LOCs={'A5','B9','A9','C1','A3','G6','E9','A6','A7','A8','B8','B1','B3','D9','B5','B4','B6','C2'}  UseAsDAC=off  DACChannel='1'  block_type=gatewayout
      settings: infoedit="Gateway out block.  Converts Xilinx fixed point inputs into ouputs of type Simulink integer, double, or fixed point.<P><P>Hardware notes:  In hardware these blocks become top level output ports or are discarded, depending on how they are configured."  xl_area=[0, 0, 0, 0, 0, 0, 0]  sginterface={'Nallatech'=>{'xdspkit'=>{'non_memory_mapped_port'=>'uprev_Shared_BRAM_addr'}},'Xilinx'=>{'jtaghwcosim'=>{'non_memory_mapped_port'=>'uprev_Shared_BRAM_addr'},'xdspkit'=>{'non_memory_mapped_port'=>'uprev_Shared_BRAM_addr'}}}
  networkanalyzer_DFTMem2_MemRecord_Shared_BRAM_data_in : xbsIndex_r4/Gateway Out  inherit_from_input=off  hdl_port=on  timing_constraint=None  locs_specified=off  LOCs={'B21','B22','A22','B23','B19','C19','A20','A21','A23','B24','A24','A25','E18','D18','C18','B18'}  UseAsDAC=off  DACChannel='1'  block_type=gatewayout
      settings: infoedit="Gateway out block.  Converts Xilinx fixed point inputs into ouputs of type Simulink integer, double, or fixed point.<P><P>Hardware notes:  In hardware these blocks become top level output ports or are discarded, depending on how they are configured."  xl_area=[0, 0, 0, 0, 0, 0, 0]  sginterface={'Nallatech'=>{'xdspkit'=>{'non_memory_mapped_port'=>'uprev_Shared_BRAM_data_in'}},'Xilinx'=>{'jtaghwcosim'=>{'non_memory_mapped_port'=>'uprev_Shared_BRAM_data_in'},'xdspkit'=>{'non_memory_mapped_port'=>'uprev_Shared_BRAM_data_in'}}}
  networkanalyzer_DFTMem2_MemRecord_Shared_BRAM_data_out : xbsIndex_r4/Gateway In  gui_display_data_type=Fixed-point  arith_type=Unsigned  n_bits=32  bin_pt=0  preci_type=Single  exp_width=8  frac_width=24  quantization=Truncate  overflow=Wrap  period=sample_rate  dbl_ovrd=off  timing_constraint=None  locs_specified=off  LOCs={}  UseAsADC=off  ADCChannel='1'  inherit_from_input=off  hdl_port=on  block_type=gatewayin
      settings: xl_area=[0, 0, 0, 0, 0, 0, 0]
  networkanalyzer_DFTMem2_MemRecord_Shared_BRAM_we : xbsIndex_r4/Gateway Out  inherit_from_input=off  hdl_port=on  timing_constraint=None  locs_specified=off  LOCs={'A14'}  UseAsDAC=off  DACChannel='1'  block_type=gatewayout
      settings: infoedit="Gateway out block.  Converts Xilinx fixed point inputs into ouputs of type Simulink integer, double, or fixed point.<P><P>Hardware notes:  In hardware these blocks become top level output ports or are discarded, depending on how they are configured."  xl_area=[0, 0, 0, 0, 0, 0, 0]
  data_out : Outport
  wires:
  convert_addr/1 -> networkanalyzer_DFTMem2_MemRecord_Shared_BRAM_addr/1
  convert_din1/1 -> networkanalyzer_DFTMem2_MemRecord_Shared_BRAM_data_in/1
  data_in/1 -> munge_in/1(din)
  calc_add/1(out) -> convert_addr/1
  networkanalyzer_DFTMem2_MemRecord_Shared_BRAM_we/1 -> mem/3(In3)
  networkanalyzer_DFTMem2_MemRecord_Shared_BRAM_data_in/1 -> mem/2(In2)
  networkanalyzer_DFTMem2_MemRecord_Shared_BRAM_addr/1 -> mem/1(In1)
  convert_we/1 -> networkanalyzer_DFTMem2_MemRecord_Shared_BRAM_we/1
  networkanalyzer_DFTMem2_MemRecord_Shared_BRAM_data_out/1 -> munge_out/1(din)
  mem/1(Out1) -> networkanalyzer_DFTMem2_MemRecord_Shared_BRAM_data_out/1
  addr/1 -> calc_add/1(in)
  we/1 -> convert_we/1
  munge_out/1(dout) -> data_out/1
  munge_in/1(dout) -> convert_din1/1
